simulink model "FiveVDC"  (Simulink 7.5)
settings: Solver=ode45  StartTime=0.0  StopTime=5  RelTol=1e-3
settings Model: Creator=lm  LastModifiedBy=lm

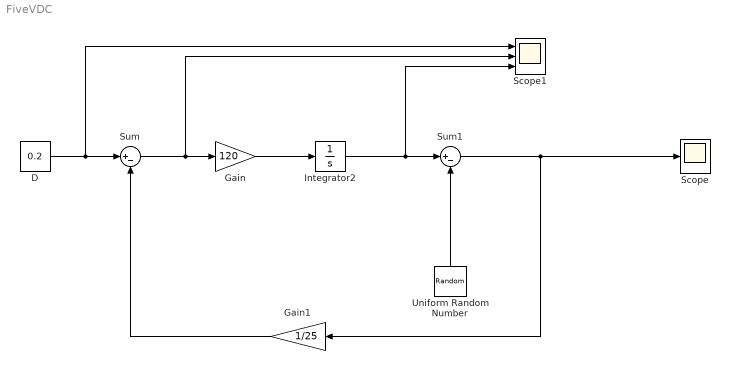
== system FiveVDC ==
  D : Constant  Value=0.2  OutDataType=fixdt(1, 16)  OutScaling=2^0
  Gain : Gain  Gain=120  ParameterDataType=fixdt(1, 16)  ParameterScaling=2^0  OutDataType=fixdt(1, 16)  OutScaling=2^0
  Gain1 : Gain  Gain=1/25  ParameterDataType=fixdt(1, 16)  ParameterScaling=2^0  OutDataType=fixdt(1, 16)  OutScaling=2^0
  Integrator2 : Integrator
  Scope : Scope
      settings: TimeRange=5  YMin=0  YMax=10
  Scope1 : Scope  NumInputPorts=3
      settings: TimeRange=5  YMin=0~-5~-5  YMax=6~5~5
  Sum : Sum  Inputs=|+-  OutDataType=fixdt(1, 16)  OutScaling=2^0
  Sum1 : Sum  Inputs=|+-  OutDataType=fixdt(1, 16)  OutScaling=2^0
  Uniform Random Number : UniformRandomNumber  Seed=10  SampleTime=0.5
  wires:
  D/1 -> Sum/1, Scope1/1
  Gain1/1 -> Sum/2
  Sum/1 -> Gain/1, Scope1/2
  Gain/1 -> Integrator2/1
  Integrator2/1 -> Sum1/1, Scope1/3
  Uniform Random Number/1 -> Sum1/2
  Sum1/1 -> Scope/1, Gain1/1
